simulink model "FOC_HSMO_G474"  (R2020b)
settings: Solver=FixedStepDiscrete  StartTime=0.0  StopTime=10  FixedStep=TsBSP  RelTol=1e-3
PreLoadFcn:
  | a=1;
undefined symbols (not defined in the file or in its folder): BandwidthCurrentPI, DiscIntNeverNeededParam, GainK, GainM, Ld, Ld_MODEL, Lq, Lq_MODEL, MaxVoltage, PolePairs, PolePairs_MODEL, PWMHalfPeriod, Rs, sigbuilder_block, TsBSP, TsFOC, TsFOC_MODEL
libraries: pid_lib x3, mcbplantlib x1, autolibpmsminterior x1
(part 2 of 2)

== system FOC_HSMO_G474/FOC/FOC_CURRENT/SVPWM/JudgeSector/If Action Subsystem/If Action Subsystem1 ==
  u_alpha_prime : Inport
  u_beta_prime : Inport  Port=2
  Action Port : ActionPort  ActionPortLabel=else
  Constant : Constant  Value=3
  Constant1 : Constant  Value=2
  Gain : Gain  Gain=-1/sqrt(3)
  Relational Operator : RelationalOperator  Operator=<  OutDataTypeStr=boolean  RndMeth=Simplest
  Switch : Switch  Criteria=u2 > Threshold
  sector : Outport
  wires:
  u_beta_prime/1 -> Gain/1
  u_alpha_prime/1 -> Relational Operator/1
  Gain/1 -> Relational Operator/2
  Relational Operator/1 -> Switch/2
  Constant/1 -> Switch/1
  Constant1/1 -> Switch/3
  Switch/1 -> sector/1

== system FOC_HSMO_G474/FOC/FOC_CURRENT/SVPWM/JudgeSector/If Action Subsystem1/If Action Subsystem ==
  u_alpha_prime : Inport
  u_beta_prime : Inport  Port=2
  Action Port : ActionPort  ActionPortLabel=if(u1)
  Constant : Constant  Value=5
  Constant1 : Constant  Value=6
  Gain : Gain  Gain=-1/sqrt(3)
  Relational Operator : RelationalOperator  Operator=<  OutDataTypeStr=boolean  RndMeth=Simplest
  Switch : Switch  Criteria=u2 > Threshold
  sector : Outport
  wires:
  u_beta_prime/1 -> Gain/1
  u_alpha_prime/1 -> Relational Operator/1
  Gain/1 -> Relational Operator/2
  Relational Operator/1 -> Switch/2
  Constant/1 -> Switch/1
  Constant1/1 -> Switch/3
  Switch/1 -> sector/1

== system FOC_HSMO_G474/FOC/FOC_CURRENT/SVPWM/JudgeSector/If Action Subsystem1/If Action Subsystem1 ==
  u_alpha_prime : Inport
  u_beta_prime : Inport  Port=2
  Action Port : ActionPort  ActionPortLabel=else
  Constant : Constant  Value=4
  Constant1 : Constant  Value=5
  Gain : Gain  Gain=1/sqrt(3)
  Relational Operator : RelationalOperator  Operator=<  OutDataTypeStr=boolean  RndMeth=Simplest
  Switch : Switch  Criteria=u2 > Threshold
  sector : Outport
  wires:
  u_beta_prime/1 -> Gain/1
  u_alpha_prime/1 -> Relational Operator/1
  Gain/1 -> Relational Operator/2
  Relational Operator/1 -> Switch/2
  Constant/1 -> Switch/1
  Constant1/1 -> Switch/3
  Switch/1 -> sector/1

== system FOC_HSMO_G474/FOC/FOC_CURRENT/HIGH_SMO/QPLL/SpeedToTheta/RangeLimit/If Action Subsystem ==
  In1 : Inport
  Action Port : ActionPort  ActionPortLabel=elseif(u2)
  Constant : Constant  Value=2*pi  OutDataTypeStr=single  SampleTime=-1
  Sum : Sum  Inputs=|++
  Out1 : Outport
  wires:
  In1/1 -> Sum/1
  Constant/1 -> Sum/2
  Sum/1 -> Out1/1

== system FOC_HSMO_G474/FOC/FOC_CURRENT/HIGH_SMO/QPLL/SpeedToTheta/RangeLimit/If Action Subsystem1 ==
  In1 : Inport
  Action Port : ActionPort  ActionPortLabel=if(u1)
  Constant : Constant  Value=2*pi  OutDataTypeStr=single  SampleTime=-1
  Sum : Sum  Inputs=|+-
  Out1 : Outport
  wires:
  In1/1 -> Sum/1
  Constant/1 -> Sum/2
  Sum/1 -> Out1/1

== system FOC_HSMO_G474/FOC/FOC_CURRENT/HIGH_SMO/QPLL/SpeedToTheta/RangeLimit/If Action Subsystem2 ==
  In1 : Inport
  Action Port : ActionPort  ActionPortLabel=else
  Out1 : Outport
  wires:
  In1/1 -> Out1/1
